simulink model "ScenarioS1"  (R2018b)
settings: Solver=VariableStepAuto  StartTime=0.0  StopTime=10  FixedStep=0.01  RelTol=1e-3  AbsTol=1e-3  EnableMultiTasking=on
libraries: sh_lib x9, fl_lib x7, nesl_utility x7
settings Model: EnablePacing=on  PacingRate=0.100000  Creator=pisaia01  LastModifiedBy=pisaia01
settings SolverCC: AutoScaleAbsTol=off
settings DataIOCC: LimitDataPoints=on  MaxDataPoints=10000
settings OptimizationCC: LifeSpan=inf
settings DebuggingCC: IgnoredZcDiagnostic=none  AllowSymbolicDim=off  LibraryContextMissingDiagnostic=none  SFUnexpectedBacktrackingDiag=warning  SFNoUnconditionalDefaultTransitionDiag=warning  SFExecutionAtInitializationDiag=none
settings SFSimCC: SimUseLocalCustomCode=off
settings RTWCC: RTWUseLocalCustomCode=off
settings CodeAppCC: StateflowObjectComments=on
settings GRTTargetCC: TargetLangStandard=C89/C90 (ANSI)  GeneratePreprocessorConditionals=Disable all
settings ConfigComp: CovMetricSettings=dw  CovHtmlReporting=on  CovSaveCumulativeToWorkspaceVar=on  CovSaveSingleToWorkspaceVar=on  CovExternalEMLEnable=off  CovSFcnEnable=off
settings SimscapeCC: SimscapeLogType=all  SimscapeLogDataHistory=10000

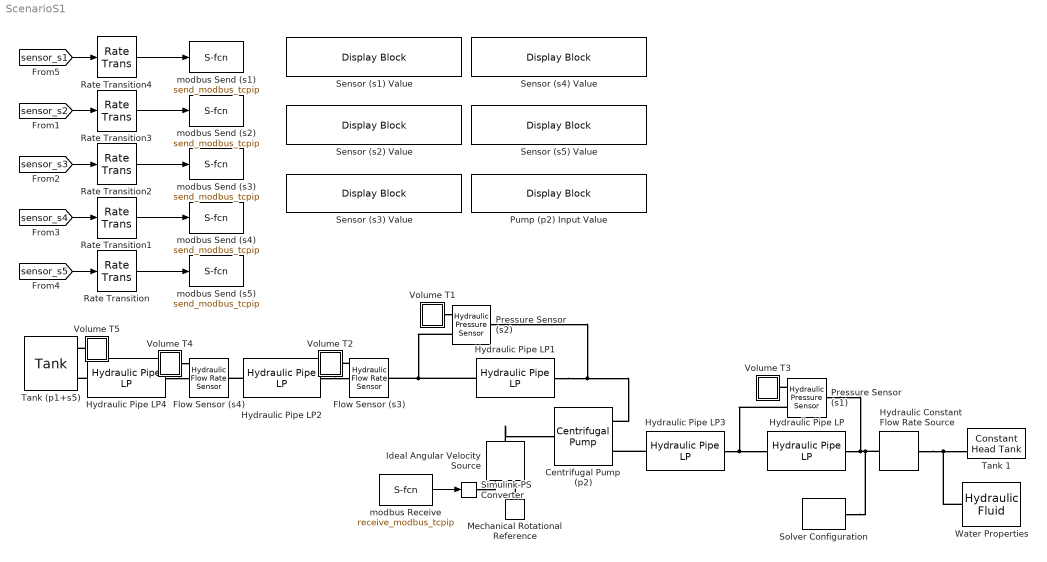
== system ScenarioS1 ==
  Centrifugal Pump (p2) : sh_lib/Pumps and Motors/Centrifugal Pump  mdl_type=1  c_1=326.8 Pa/(kg/m^3)  c_2=3.104e4 Pa*s/kg  c_3=1.097e7 Pa*s^2/(kg*m^3)  c_4=2.136e5 Pa*s^2/(kg*m^3)  c_f=0.8  design_del=130 lpm  ref_velocity=1770 rpm  ref_density=920 kg/m^3  leak_resistance=1e8 Pa/(m^3/s)  T_const=0.1 N*m  trq_press_coeff=0.1e-5 N*m/Pa  pump_del_1D=[0, 28, 90, 130, 154, 182] lpm  press_diff_1D=[2.6, 2.4, 2, 1.6, 1.2, .8] bar  pump_del_power_1D=[0, 20, 40, 60, 80, 100, 120, 140, 160] lpm  power_1D=[220, 280, 310, 360, 390, 420, 480, 500, 550] W  pump_vel_2D=[3200, 3300, 3400, 3500] rpm  pump_del_2D=[0, 50, 100, 150, 200, 250, 300, 350] lpm  press_diff_2D=[8.3, 8.8, 9.3, 9.9; 7.8, 8.3, 8.8, 9.4; 7.2, 7.6, 8.2, 8.7; 6.5, 7, 7.5, 8; 5.6, 6.1, 6.6, 7.1; 4.7, 5.2, 5.7, 6.2; 3.4, 4, 4.4, 4.9; 2.3, 2.7, 3.4, 3.6] bar  pump_del_power_2D=[0, 50, 100, 150, 200, 250, 300, 350] lpm  power_2D=[1223, 1341, 1467, 1600; 1414, 1551, 1696, 1850; 1636, 1794, 1962, 2140; 1941, 2129, 2326, 2540; 2224, 2439, 2660, 2910; 2453, 2691, 2947, 3210; 2757, 3024, 3307, 3608; 2945, 3230, 3533, 3854] W  omega_threshold=1e-9 rad/s  interp_method=1  extrap_method=1
      settings: SourceProductName=Simscape Fluids  SourceProductBaseCode=SH
  Flow Sensor (s3) : fl_lib/Hydraulic/Hydraulic Sensors/Hydraulic Flow Rate Sensor
      settings: SourceProductName=Simscape
  Flow Sensor (s4) : fl_lib/Hydraulic/Hydraulic Sensors/Hydraulic Flow Rate Sensor
      settings: SourceProductName=Simscape
  Hydraulic Constant Flow Rate Source : fl_lib/Hydraulic/Hydraulic Sources/Hydraulic Constant Flow Rate Source  commanded_flow_rate=10 m^3/s
      settings: SourceProductName=Simscape  SourceProductBaseCode=SS
  Hydraulic Pipe LP{,1..4} (5 alike) : sh_lib/Low-Pressure Blocks/Hydraulic Pipe LP  cs_type=1  d_in=300 mm  area=1e-4 m^2  D_h=1.12e-2 m  s_factor=64  length=5 m  length_ad=1 m  roughness=15e-6 m  Re_lam=2000  Re_turb=4000  elevation_A=0 m  elevation_B=0 m  g=9.80665 m/s^2  wall_type=1  pr_r_coef=2e-12 m/Pa  time_const=0.01 s  k_sh=1.4  p0=0 Pa
      settings: SourceProductName=Simscape Fluids  SourceProductBaseCode=SH
  Ideal Angular Velocity Source : fl_lib/Mechanical/Mechanical Sources/Ideal Angular Velocity Source
  Mechanical Rotational Reference : fl_lib/Mechanical/Rotational Elements/Mechanical Rotational Reference
  Pressure Sensor (s1) : fl_lib/Hydraulic/Hydraulic Sensors/Hydraulic Pressure Sensor
      settings: SourceProductName=Simscape
  Pressure Sensor (s2) : fl_lib/Hydraulic/Hydraulic Sensors/Hydraulic Pressure Sensor
      settings: SourceProductName=Simscape
  Pump (p2) Input Value : DisplayBlock  WebBlockId=225  LabelPosition=Hide
  Rate Transition{,1..3} (4 alike) : RateTransition  OutPortSampleTime=0.01
  Rate Transition4 : RateTransition  OutPortSampleTime=0.05
  Sensor (s1) Value : DisplayBlock  WebBlockId=226  LabelPosition=Hide
  Sensor (s2) Value : DisplayBlock  WebBlockId=227  LabelPosition=Hide
  Sensor (s3) Value : DisplayBlock  WebBlockId=228  LabelPosition=Hide
  Sensor (s4) Value : DisplayBlock  WebBlockId=229  LabelPosition=Hide
  Sensor (s5) Value : DisplayBlock  WebBlockId=230  LabelPosition=Hide
  Simulink-PS Converter : nesl_utility/Simulink-PS Converter  PhysicalDomain=network_engine_domain  SubClassName=ps_input  LeftPortType=input  RightPortType=output  PseudoPeriodic=off  Frequencies=[]  NoiseDistribution=none  NoiseParameters=[]  Unit=1  AffineConversion=off  FilteringAndDerivatives=provide  SimscapeFilterOrder=1  InputFilterTimeConstant=0.001  UdotUserProvided=0
  Solver Configuration : nesl_utility/Solver Configuration  PhysicalDomain=network_engine_domain  SubClassName=solver  LeftPortType=input  RightPortType=generic  Tones=[]  Harmonics=[]  SimulateNoise=off  Profile=off  UseLocalSampling=off  EnableSwitchedLinearOptims=on  FrequencyDomain=off  UseCCode=off  RelTol=0.001  AbsTol=1e-06  MinStep=1e-09  ToWorkspace=off  RevertToSquareIcSolve=off  NumHomotopyIterations=100  PhasorMode=off  PhasorModeNumHarmonics=1  DoDC=off  ResidualTolerance=1e-09  UseLocalSolver=off  LocalSolverChoice=NE_BACKWARD_EULER_ADVANCER  LocalSolverSampleTime=0.001  DoFixedCost=off  MaxNonlinIter=3  MaxModeIter=2  LinearAlgebra=auto  EquationFormulation=NE_TIME_EF  DelaysMemoryBudget=1024  AutomaticFiltering=on  FilteringTimeConstant=0.001  PartitionStorageMethod=AS_NEEDED  PartitionMemoryBudget=1024
  Tank (p1+s5) : sh_lib/Low-Pressure Blocks/Tank  press=0 Pa  level_spec=1  tank_area=0.8 m^2  fluid_volume_tab=[0, .0028, .0065, .0114, .0176, .0252, .0344, .0436, .0512, .0574, .0623, .066, .0688, .0707, .072, .0727] m^3  fluid_level_tab=[0, .02, .04, .06, .08, .1, .12, .14, .16, .18, .2, .22, .24, .26, .28, .3] m  interp_method=1  extrap_method=1  pipe_diam=0.02 m  loss_coeff=1.2  g=9.80665 m/s^2  min_level=1e-3 m  fluid_level_check=0  volume_specify=off  volume_priority=High  volume=20 l  volume_nominal_specify=off  volume_nominal_unit=l  volume_nominal_value=1  level_specify=off  level_priority=None  level=0.025 m  level_nominal_specify=off  level_nominal_unit=m  level_nominal_value=1  pipe_diam_A=0.02 m  loss_coeff_A=1.2  height_B=0.8 m  pipe_diam_B=0.02 m  loss_coeff_B=1.2  height_C=0.8 m  pipe_diam_C=0.02 m  loss_coeff_C=1.2
      settings: SourceProductName=Simscape Fluids  SourceProductBaseCode=SH
  Tank 1 : sh_lib/Low-Pressure Blocks/Constant Head Tank  press=0 Pa  fluid_level=200 m  pipe_diam=0.02 m  loss_coeff=1.2  g=9.80665 m/s^2  volume_specify=on  volume_priority=High  volume=15 m^3  volume_nominal_specify=off  volume_nominal_unit=m^3  volume_nominal_value=1
      settings: SourceProductName=Simscape Fluids  SourceProductBaseCode=SH
  Volume T1 : Subsystem
  Volume T2 : Subsystem
  Volume T3 : Subsystem
  Volume T4 : Subsystem
  Volume T5 : Subsystem
  Water Properties : sh_lib/Hydraulic Utilities/Hydraulic Fluid  DataSource=1  SelFluid=24  SysTemp=30  TrapAir=0.001  ViscDerFactor=1  range_error=2
      settings: SourceProductName=Simscape Fluids
  modbus Receive : M-S-Function  FunctionName=receive_modbus_tcpip  Parameters=40
  modbus Send (s1) : M-S-Function  FunctionName=send_modbus_tcpip  Parameters=0
  modbus Send (s2) : M-S-Function  FunctionName=send_modbus_tcpip  Parameters=8
  modbus Send (s3) : M-S-Function  FunctionName=send_modbus_tcpip  Parameters=16
  modbus Send (s4) : M-S-Function  FunctionName=send_modbus_tcpip  Parameters=24
  modbus Send (s5) : M-S-Function  FunctionName=send_modbus_tcpip  Parameters=32
  wires:
  [sensor_s1] -> Rate Transition4/1
  [sensor_s2] -> Rate Transition3/1
  [sensor_s3] -> Rate Transition2/1
  [sensor_s4] -> Rate Transition1/1
  [sensor_s5] -> Rate Transition/1
  Rate Transition4/1 -> modbus Send (s1)/1
  Rate Transition3/1 -> modbus Send (s2)/1
  Rate Transition2/1 -> modbus Send (s3)/1
  Rate Transition1/1 -> modbus Send (s4)/1
  Rate Transition/1 -> modbus Send (s5)/1
  modbus Receive/1 -> Simulink-PS Converter/1
  connections:
  Ideal Angular Velocity Source/LConn1 -- Centrifugal Pump (p2)/LConn1
  Mechanical Rotational Reference/LConn1 -- Ideal Angular Velocity Source/RConn2
  Simulink-PS Converter/RConn1 -- Ideal Angular Velocity Source/RConn1
  Hydraulic Constant Flow Rate Source/LConn1 -- Solver Configuration/RConn1 -- Pressure Sensor (s1)/LConn1 -- Hydraulic Pipe LP/LConn1
  Hydraulic Pipe LP2/RConn1 -- Flow Sensor (s4)/LConn1
  Hydraulic Pipe LP4/RConn1 -- Tank (p1+s5)/RConn2
  Hydraulic Pipe LP4/LConn1 -- Flow Sensor (s4)/RConn2
  Hydraulic Constant Flow Rate Source/RConn1 -- Water Properties/RConn1 -- Tank 1/RConn2
  Hydraulic Pipe LP3/RConn1 -- Centrifugal Pump (p2)/RConn2
  Hydraulic Pipe LP2/LConn1 -- Flow Sensor (s3)/RConn2
  Hydraulic Pipe LP3/LConn1 -- Hydraulic Pipe LP/RConn1 -- Pressure Sensor (s1)/RConn1
  Hydraulic Pipe LP1/RConn1 -- Pressure Sensor (s2)/RConn1 -- Flow Sensor (s3)/LConn1
  Hydraulic Pipe LP1/LConn1 -- Pressure Sensor (s2)/LConn1 -- Centrifugal Pump (p2)/RConn1
  Pressure Sensor (s1)/RConn2 -- Volume T3/LConn1
  Volume T1/LConn1 -- Pressure Sensor (s2)/RConn2
  Flow Sensor (s3)/RConn1 -- Volume T2/LConn1
  Volume T4/LConn1 -- Flow Sensor (s4)/RConn1
  Volume T5/LConn1 -- Tank (p1+s5)/RConn1

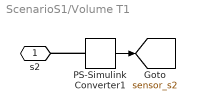
== system ScenarioS1/Volume T1 ==
  PS-Simulink Converter1 : nesl_utility/PS-Simulink Converter  PhysicalDomain=network_engine_domain  SubClassName=ps_output  LeftPortType=input  RightPortType=output  PseudoPeriodic=off  Frequencies=[]  Unit=1  AffineConversion=off
  s2 : PMIOPort  Side=Left
  tag scope: sensor_s2=global
  wires:
  PS-Simulink Converter1/1 -> [sensor_s2]
  connections:
  PS-Simulink Converter1/LConn1 -- s2/RConn1

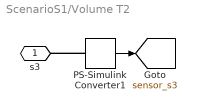
== system ScenarioS1/Volume T2 ==
  PS-Simulink Converter1 : nesl_utility/PS-Simulink Converter  PhysicalDomain=network_engine_domain  SubClassName=ps_output  LeftPortType=input  RightPortType=output  PseudoPeriodic=off  Frequencies=[]  Unit=1  AffineConversion=off
  s3 : PMIOPort  Side=Left
  tag scope: sensor_s3=global
  wires:
  PS-Simulink Converter1/1 -> [sensor_s3]
  connections:
  PS-Simulink Converter1/LConn1 -- s3/RConn1

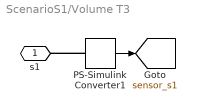
== system ScenarioS1/Volume T3 ==
  PS-Simulink Converter1 : nesl_utility/PS-Simulink Converter  PhysicalDomain=network_engine_domain  SubClassName=ps_output  LeftPortType=input  RightPortType=output  PseudoPeriodic=off  Frequencies=[]  Unit=1  AffineConversion=off
  s1 : PMIOPort  Side=Left
  tag scope: sensor_s1=global
  wires:
  PS-Simulink Converter1/1 -> [sensor_s1]
  connections:
  PS-Simulink Converter1/LConn1 -- s1/RConn1

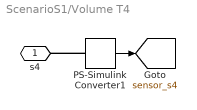
== system ScenarioS1/Volume T4 ==
  PS-Simulink Converter1 : nesl_utility/PS-Simulink Converter  PhysicalDomain=network_engine_domain  SubClassName=ps_output  LeftPortType=input  RightPortType=output  PseudoPeriodic=off  Frequencies=[]  Unit=1  AffineConversion=off
  s4 : PMIOPort  Side=Left
  tag scope: sensor_s4=global
  wires:
  PS-Simulink Converter1/1 -> [sensor_s4]
  connections:
  PS-Simulink Converter1/LConn1 -- s4/RConn1

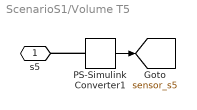
== system ScenarioS1/Volume T5 ==
  PS-Simulink Converter1 : nesl_utility/PS-Simulink Converter  PhysicalDomain=network_engine_domain  SubClassName=ps_output  LeftPortType=input  RightPortType=output  PseudoPeriodic=off  Frequencies=[]  Unit=1  AffineConversion=off
  s5 : PMIOPort  Side=Left
  tag scope: sensor_s5=global
  wires:
  PS-Simulink Converter1/1 -> [sensor_s5]
  connections:
  PS-Simulink Converter1/LConn1 -- s5/RConn1
